simulink model "non_linear_damped_pendulum"  (R2024a)
settings: Solver=FixedStepAuto  StartTime=0.0  StopTime=40  FixedStep=1e-3  RelTol=1e-3
InitFcn:
  | J = 0.4; % [kg*m^2]
  | c = 0.2; % damping factor
  | m = 0.4; % [kg]
  | g = 9.8; % [m/s^2]
  | d = 0.05; % [m]
  | r = 0.4; % [m]
libraries: simulink_extras x1
settings Model: Creator=toninho  LastModifiedBy=toninho

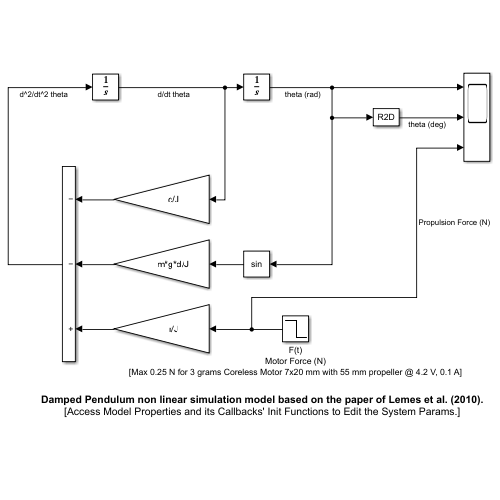
[thumbnail: Simulink's stored preview of the top-level diagram]
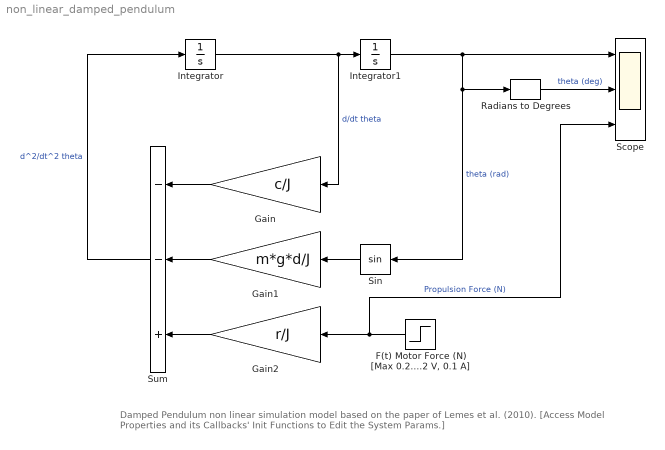
== system non_linear_damped_pendulum ==
  note: Damped Pendulum non linear simulation model based on the paper of Lemes et al. (2010).
      | [Access Model Properties and its Callbacks' Init Functions to Edit the System Params.]
  "F(t) Motor Force (N) [Max 0.25 N for 3 grams Coreless Motor 7x20 mm with 55 mm propeller @ 4.2 V, 0.1 A]" : Step  Time=20  Before=0.25/1  After=0.25/2  SampleTime=0
  Gain : Gain  Gain=c/J
  Gain1 : Gain  Gain=m*g*d/J
  Gain2 : Gain  Gain=r/J
  Integrator : Integrator
  Integrator1 : Integrator
  Radians to Degrees : simulink_extras/Transformations/Radians to Degrees
  Scope : Scope  NumInputPorts=3
  Sin : Trigonometry  OutputSignalType=real
  Sum : Sum  Inputs=--+
  wires:
  Integrator/1 -> Gain/1, Integrator1/1  "d/dt theta"
  Integrator1/1 -> Scope/1, Radians to Degrees/1, Sin/1  "theta (rad)"
  Gain/1 -> Sum/1
  Gain1/1 -> Sum/2
  Gain2/1 -> Sum/3
  Sum/1 -> Integrator/1  "d^2/dt^2 theta"
  "F(t) Motor Force (N) [Max 0.25 N for 3 grams Coreless Motor 7x20 mm with 55 mm propeller @ 4.2 V, 0.1 A]"/1 -> Scope/3, Gain2/1  "Propulsion Force (N)"
  Sin/1 -> Gain1/1
  Radians to Degrees/1 -> Scope/2  "theta (deg)"
